simulink model "Assignment1"  (R2017a)
settings: Solver=FixedStepAuto  StartTime=0.0  StopTime=10.0  FixedStep=1E-3  RelTol=1e-3  EnableMultiTasking=on
undefined symbols (not defined in the file): D0, D1, D10, D11, D12, D13, D2, D3, D4, D5, D6, D7, D8, D9, PTA0, PTA1, PTA2, PTB23, PTB9, PTC16, PTC17, PTC2, PTC3, PTC4, PTD0, PTD1, PTD2, PTD3
libraries: frdmk64flib x18
settings Model: ExtModeTrigDuration=5  Creator=Nathe  LastModifiedBy=Nathe
settings DataIOCC: ReturnWorkspaceOutputs=on
settings OptimizationCC: EnhancedBackFolding=on  PassReuseOutputArgsAs=Individual arguments  ZeroExternalMemoryAtStartup=off  ZeroInternalMemoryAtStartup=off  MaxStackSize=64  OptimizeBlockOrder=speed
settings DebuggingCC: ParameterTunabilityLossMsg=error
settings HardwareCC: ProdBitPerPointer=32  ProdBitPerSizeT=32  ProdBitPerPtrDiffT=32  ProdLargestAtomicInteger=Long  ProdLargestAtomicFloat=Double  ProdWordSize=32  ProdHWDeviceType=ARM Compatible->ARM Cortex
settings SFSimCC: SimUseLocalCustomCode=on  MATLABDynamicMemAlloc=off
settings RTWCC: SystemTargetFile=ert.tlc  HardwareBoard=NXP FRDM-K64F  TLCOptions="-aInlineSetEventsForThisBaseRateFcn=TLC_FALSE -aSuppressMultiTaskScheduler=TLC_FALSE  -aRateBasedStepFcn=0"  TemplateMakefile=ert_default_tmf  Description=Embedded Coder  GenerateReport=on  RTWUseLocalCustomCode=on  Toolchain=GNU Tools for ARM Embedded Processors  IncludeHyperlinkInReport=on  LaunchReport=on  GenerateTraceInfo=on  GenerateTraceReport=on  GenerateTraceReportSl=on  GenerateTraceReportSf=on  GenerateTraceReportEml=on
settings CodeAppCC: ForceParamTrailComments=on  IgnoreCustomStorageClasses=off  OperatorAnnotations=on  SimulinkDataObjDesc=on  SFDataObjDesc=on  InsertBlockDesc=on
settings ERTTargetCC: SupportContinuousTime=on
settings SimscapeCC: SelectedTab=General

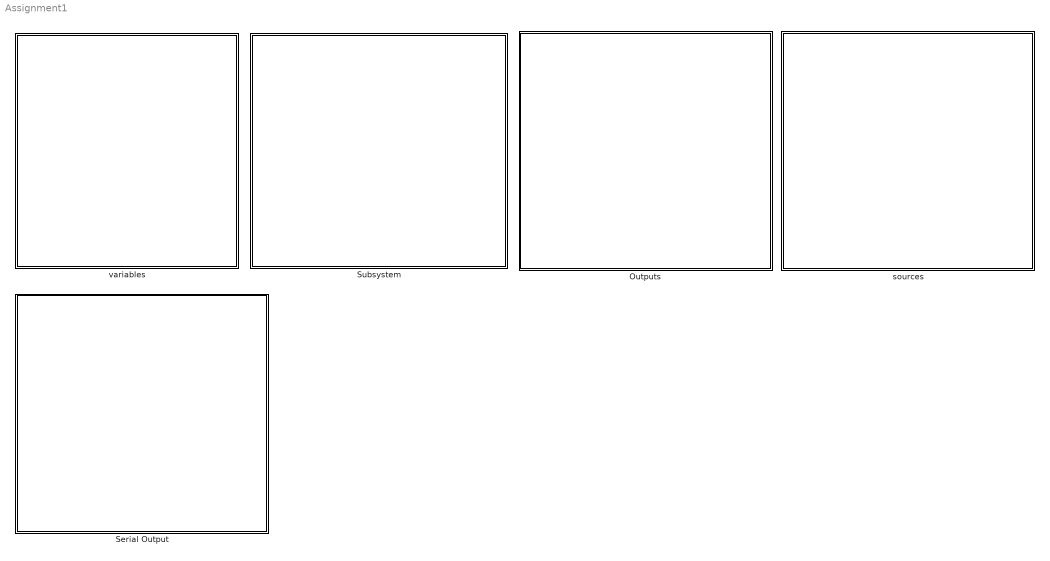
== system Assignment1 ==
  "Outputs " : Subsystem
  Serial Output : Subsystem
  Subsystem : Subsystem
  "sources " : Subsystem
  "variables " : Subsystem

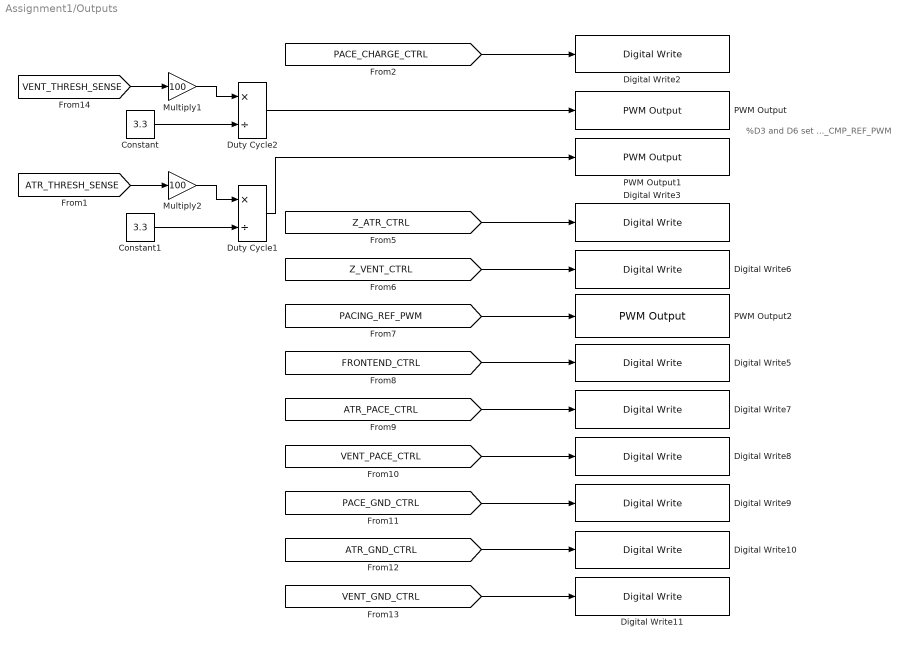
== system Assignment1/Outputs  ==
  note: %D3 and D6 set ..._CMP_REF_PWM
  Constant : Constant  Value=3.3
  Constant1 : Constant  Value=3.3
  Digital Write10 : frdmk64flib/Digital Write  Whichpin=PTD2 (D11)
      settings: SourceProductName=Simulink Coder Support Package for NXP FRDM-K64F Board
  Digital Write11 : frdmk64flib/Digital Write  Whichpin=PTD3 (D12)
      settings: SourceProductName=Simulink Coder Support Package for NXP FRDM-K64F Board
  Digital Write2 : frdmk64flib/Digital Write  Whichpin=PTB9 (D2)
      settings: SourceProductName=Simulink Coder Support Package for NXP FRDM-K64F Board
  Digital Write3 : frdmk64flib/Digital Write  Whichpin=PTB23 (D4)
      settings: SourceProductName=Simulink Coder Support Package for NXP FRDM-K64F Board
  Digital Write5 : frdmk64flib/Digital Write  Whichpin=PTD1 (D13)
      settings: SourceProductName=Simulink Coder Support Package for NXP FRDM-K64F Board
  Digital Write6 : frdmk64flib/Digital Write  Whichpin=PTC3 (D7)
      settings: SourceProductName=Simulink Coder Support Package for NXP FRDM-K64F Board
  Digital Write7 : frdmk64flib/Digital Write  Whichpin=PTA0 (D8)
      settings: SourceProductName=Simulink Coder Support Package for NXP FRDM-K64F Board
  Digital Write8 : frdmk64flib/Digital Write  Whichpin=PTC4 (D9)
      settings: SourceProductName=Simulink Coder Support Package for NXP FRDM-K64F Board
  Digital Write9 : frdmk64flib/Digital Write  Whichpin=PTD0 (D10)
      settings: SourceProductName=Simulink Coder Support Package for NXP FRDM-K64F Board
  Duty Cycle1 : Product  Inputs=*/  SaturateOnIntegerOverflow=off  RndMeth=Floor  InputSameDT=off  OutDataTypeStr=Inherit: Inherit via internal rule
  Duty Cycle2 : Product  Inputs=*/  SaturateOnIntegerOverflow=off  RndMeth=Floor  InputSameDT=off  OutDataTypeStr=Inherit: Inherit via internal rule
  Multiply1 : Gain  Gain=100
  Multiply2 : Gain  Gain=100
  PWM Output : frdmk64flib/PWM Output  Whichpin=PTA1 (D3)  InitialFrequency=2000  InitialDutyCycle=0
      settings: SourceProductName=Simulink Coder Support Package for NXP FRDM-K64F Board
  PWM Output1 : frdmk64flib/PWM Output  Whichpin=PTC2 (D6)  InitialFrequency=2000  InitialDutyCycle=0
      settings: SourceProductName=Simulink Coder Support Package for NXP FRDM-K64F Board
  PWM Output2 : frdmk64flib/PWM Output  Whichpin=PTA2 (D5)  InitialFrequency=2000  InitialDutyCycle=0
      settings: SourceProductName=Simulink Coder Support Package for NXP FRDM-K64F Board
  wires:
  [PACING_REF_PWM] -> PWM Output2/1
  [VENT_GND_CTRL] -> Digital Write11/1
  [PACE_GND_CTRL] -> Digital Write9/1
  [FRONTEND_CTRL] -> Digital Write5/1
  [VENT_PACE_CTRL] -> Digital Write8/1
  [ATR_PACE_CTRL] -> Digital Write7/1
  [Z_VENT_CTRL] -> Digital Write6/1
  [ATR_GND_CTRL] -> Digital Write10/1
  [PACE_CHARGE_CTRL] -> Digital Write2/1
  Duty Cycle2/1 -> PWM Output/1
  [Z_ATR_CTRL] -> Digital Write3/1
  [VENT_THRESH_SENSE] -> Multiply1/1
  Duty Cycle1/1 -> PWM Output1/1
  Constant1/1 -> Duty Cycle1/2
  Constant/1 -> Duty Cycle2/2
  [ATR_THRESH_SENSE] -> Multiply2/1
  Multiply1/1 -> Duty Cycle2/1
  Multiply2/1 -> Duty Cycle1/1

== system Assignment1/Serial Output ==

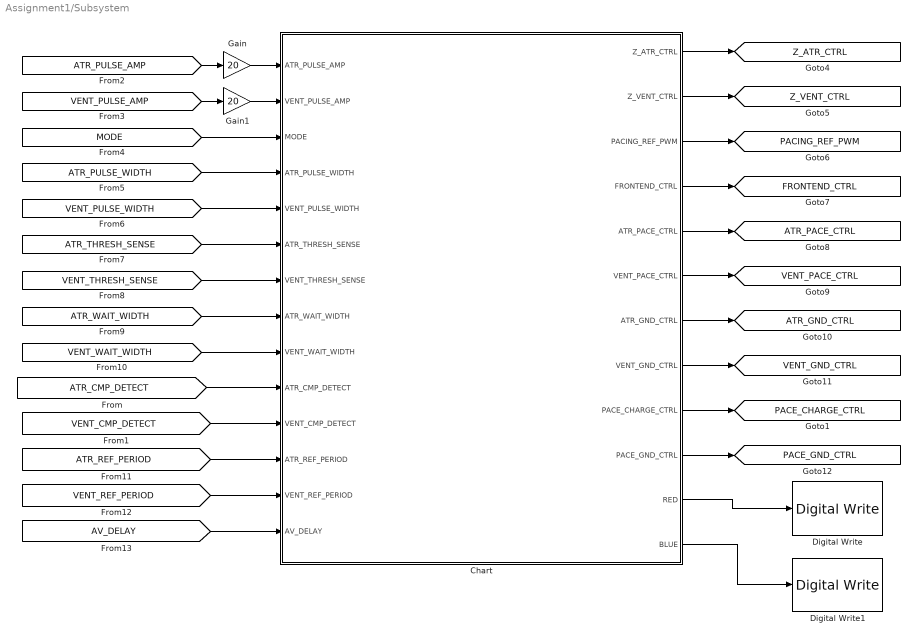
== system Assignment1/Subsystem ==
  Chart : Stateflow chart  TreatAsAtomicUnit=on
  Digital Write : frdmk64flib/Digital Write  Whichpin=RED_LED
      settings: SourceProductName=Simulink Coder Support Package for NXP FRDM-K64F Board
  Digital Write1 : frdmk64flib/Digital Write  Whichpin=BLUE_LED
      settings: SourceProductName=Simulink Coder Support Package for NXP FRDM-K64F Board
  Gain : Gain  Gain=20
  Gain1 : Gain  Gain=20
  tag scope: ATR_GND_CTRL=global, ATR_PACE_CTRL=global, FRONTEND_CTRL=global, PACE_CHARGE_CTRL=global, PACE_GND_CTRL=global, PACING_REF_PWM=global, VENT_GND_CTRL=global, VENT_PACE_CTRL=global, Z_ATR_CTRL=global, Z_VENT_CTRL=global
  wires:
  [ATR_CMP_DETECT] -> Chart/10(ATR_CMP_DETECT)
  Gain/1 -> Chart/1(ATR_PULSE_AMP)
  Chart/3(PACING_REF_PWM) -> [PACING_REF_PWM]
  Chart/7(ATR_GND_CTRL) -> [ATR_GND_CTRL]
  [VENT_WAIT_WIDTH] -> Chart/9(VENT_WAIT_WIDTH)
  Chart/2(Z_VENT_CTRL) -> [Z_VENT_CTRL]
  Chart/5(ATR_PACE_CTRL) -> [ATR_PACE_CTRL]
  [VENT_PULSE_WIDTH] -> Chart/5(VENT_PULSE_WIDTH)
  [ATR_PULSE_AMP] -> Gain/1
  Chart/9(PACE_CHARGE_CTRL) -> [PACE_CHARGE_CTRL]
  [ATR_PULSE_WIDTH] -> Chart/4(ATR_PULSE_WIDTH)
  Chart/8(VENT_GND_CTRL) -> [VENT_GND_CTRL]
  Chart/1(Z_ATR_CTRL) -> [Z_ATR_CTRL]
  [VENT_PULSE_AMP] -> Gain1/1
  [VENT_THRESH_SENSE] -> Chart/7(VENT_THRESH_SENSE)
  [VENT_CMP_DETECT] -> Chart/11(VENT_CMP_DETECT)
  Chart/4(FRONTEND_CTRL) -> [FRONTEND_CTRL]
  Chart/6(VENT_PACE_CTRL) -> [VENT_PACE_CTRL]
  [MODE] -> Chart/3(MODE)
  [ATR_THRESH_SENSE] -> Chart/6(ATR_THRESH_SENSE)
  [ATR_WAIT_WIDTH] -> Chart/8(ATR_WAIT_WIDTH)
  Gain1/1 -> Chart/2(VENT_PULSE_AMP)
  Chart/10(PACE_GND_CTRL) -> [PACE_GND_CTRL]
  Chart/11(RED) -> Digital Write/1
  Chart/12(BLUE) -> Digital Write1/1
  [ATR_REF_PERIOD] -> Chart/12(ATR_REF_PERIOD)
  [VENT_REF_PERIOD] -> Chart/13(VENT_REF_PERIOD)
  [AV_DELAY] -> Chart/14(AV_DELAY)

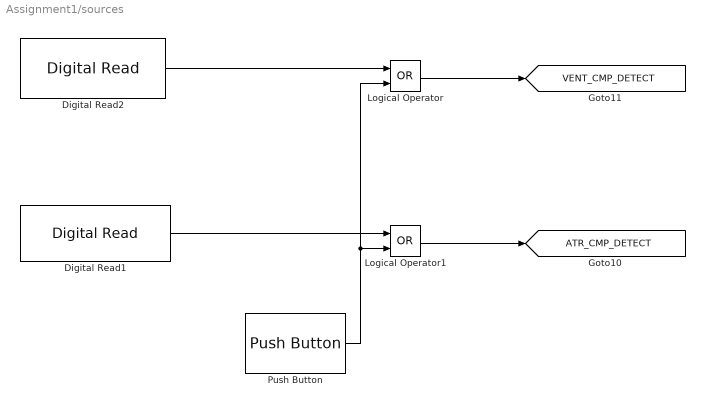
== system Assignment1/sources  ==
  Digital Read1 : frdmk64flib/Digital Read  Whichpin=PTC16 (D0)  SampleTime=-1
      settings: SourceProductName=Simulink Coder Support Package for NXP FRDM-K64F Board
  Digital Read2 : frdmk64flib/Digital Read  Whichpin=PTC17 (D1)  SampleTime=-1
      settings: SourceProductName=Simulink Coder Support Package for NXP FRDM-K64F Board
  Logical Operator : Logic  Operator=OR  AllPortsSameDT=off  OutDataTypeStr=boolean
  Logical Operator1 : Logic  Operator=OR  AllPortsSameDT=off  OutDataTypeStr=boolean
  Push Button : frdmk64flib/Push Button  Whichswitch=SW2  SampleTime1=-1
      settings: SourceProductName=Simulink Coder Support Package for NXP FRDM-K64F Board
  tag scope: ATR_CMP_DETECT=global, VENT_CMP_DETECT=global
  wires:
  Digital Read2/1 -> Logical Operator/1
  Logical Operator/1 -> [VENT_CMP_DETECT]
  Digital Read1/1 -> Logical Operator1/1
  Logical Operator1/1 -> [ATR_CMP_DETECT]
  Push Button/1 -> Logical Operator/2, Logical Operator1/2

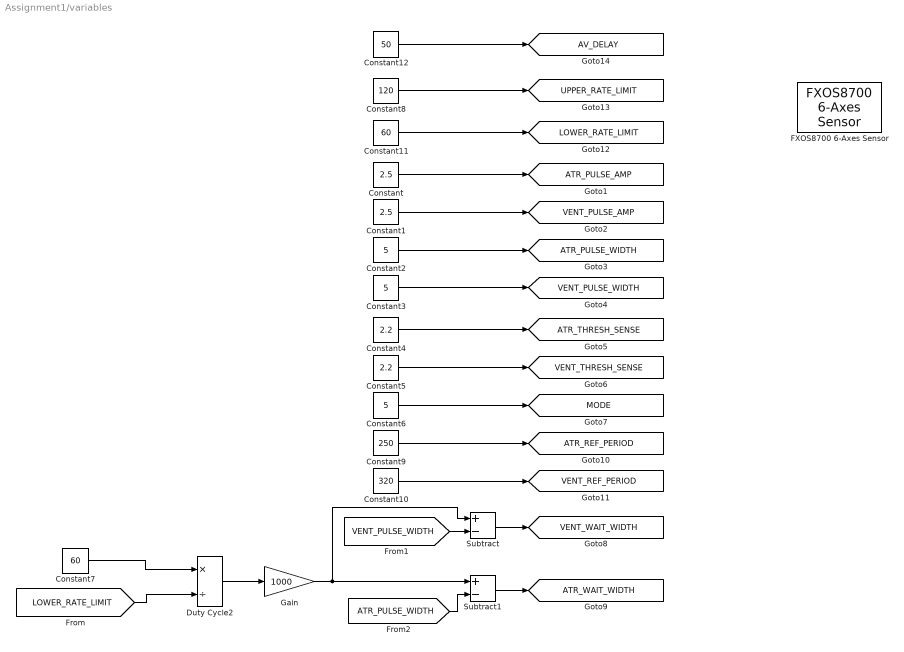
== system Assignment1/variables  ==
  Constant : Constant  Value=2.5
  Constant1 : Constant  Value=2.5
  Constant10 : Constant  Value=320
  Constant11 : Constant  Value=60
  Constant12 : Constant  Value=50
  Constant2 : Constant  Value=5
  Constant3 : Constant  Value=5
  Constant4 : Constant  Value=2.2
  Constant5 : Constant  Value=2.2
  Constant6 : Constant  Value=5  OutDataTypeStr=int8
  Constant7 : Constant  Value=60
  Constant8 : Constant  Value=120
  Constant9 : Constant  Value=250
  Duty Cycle2 : Product  Inputs=*/  SaturateOnIntegerOverflow=off  RndMeth=Floor  InputSameDT=off  OutDataTypeStr=Inherit: Inherit via internal rule
  FXOS8700 6-Axes Sensor : frdmk64flib/FXOS8700 6-Axes Sensor  Activesensor=Accelerometer only  ODR=800Hz  HybridODR=400Hz  Accelfullrange=-4g to +4g  SampleTime=-1
      settings: SourceProductName=Simulink Coder Support Package for NXP FRDM-K64F Board
  Gain : Gain  Gain=1000
  Subtract : Sum  Inputs=+-  SaturateOnIntegerOverflow=off  InputSameDT=off  OutDataTypeStr=Inherit: Inherit via internal rule
  Subtract1 : Sum  Inputs=+-  SaturateOnIntegerOverflow=off  InputSameDT=off  OutDataTypeStr=Inherit: Inherit via internal rule
  tag scope: ATR_PULSE_AMP=global, ATR_PULSE_WIDTH=global, ATR_REF_PERIOD=global, ATR_THRESH_SENSE=global, ATR_WAIT_WIDTH=global, AV_DELAY=global, LOWER_RATE_LIMIT=global, MODE=global, UPPER_RATE_LIMIT=global, VENT_PULSE_AMP=global, VENT_PULSE_WIDTH=global, VENT_REF_PERIOD=global, VENT_THRESH_SENSE=global, VENT_WAIT_WIDTH=global
  wires:
  Constant3/1 -> [VENT_PULSE_WIDTH]
  Constant2/1 -> [ATR_PULSE_WIDTH]
  Constant/1 -> [ATR_PULSE_AMP]
  Constant5/1 -> [VENT_THRESH_SENSE]
  Constant1/1 -> [VENT_PULSE_AMP]
  Constant4/1 -> [ATR_THRESH_SENSE]
  Constant6/1 -> [MODE]
  Subtract/1 -> [VENT_WAIT_WIDTH]
  Subtract1/1 -> [ATR_WAIT_WIDTH]
  Constant9/1 -> [ATR_REF_PERIOD]
  Constant10/1 -> [VENT_REF_PERIOD]
  Constant11/1 -> [LOWER_RATE_LIMIT]
  Constant7/1 -> Duty Cycle2/1
  [LOWER_RATE_LIMIT] -> Duty Cycle2/2
  Duty Cycle2/1 -> Gain/1
  Gain/1 -> Subtract1/1, Subtract/1
  [VENT_PULSE_WIDTH] -> Subtract/2
  [ATR_PULSE_WIDTH] -> Subtract1/2
  Constant8/1 -> [UPPER_RATE_LIMIT]
  Constant12/1 -> [AV_DELAY]

== stateflow chart Assignment1/Subsystem/Chart ==
  state AAIR [group]
    state CHARGEC22_DISCHARGEC21
      during:
      %CHARGE C22
      PACING_REF_PWM = ATR_PULSE_AMP
      PACE_CHARGE_CTRL = true
      ATR_PACE_CTRL = false
      VENT_PACE_CTRL = false
      %DISCHARGE C21
      PACE_GND_CTRL = true
      VENT_PACE_CTRL = false
      VENT_GND_CTRL = false
      ATR_GND_CTRL = true
      RED = false
      BLUE = false
      Z_ATR_CTRL=false
      Z_VENT_CTRL=false
      FRONTEND_CTRL=true
    state DISCHARGEC22
      %paces atrium
      during:
      %CHARGE C21
      ATR_PACE_CTRL = true
      PACE_CHARGE_CTRL = false
      ATR_GND_CTRL = false
      PACE_GND_CTRL = true
      VENT_PACE_CTRL = false
      VENT_GND_CTRL = false
      Z_ATR_CTRL=false
      Z_VENT_CTRL=false
      FRONTEND_CTRL=true
      RED = true
    state CHARGEC22_DISCHARGEC21_2
      during:
      %CHARGE C22
      PACING_REF_PWM = ATR_PULSE_AMP
      PACE_CHARGE_CTRL = true
      ATR_PACE_CTRL = false
      VENT_PACE_CTRL = false
      %DISCHARGE C21
      PACE_GND_CTRL = true
      VENT_PACE_CTRL = false
      VENT_GND_CTRL = false
      ATR_GND_CTRL = true
      RED = false
      BLUE = false
      Z_ATR_CTRL=false
      Z_VENT_CTRL=false
      FRONTEND_CTRL=true
    state DUMMY
      during:
      BLUE = true
      RED = false
    AAIR.CHARGEC22_DISCHARGEC21 -> AAIR.DISCHARGEC22 [order 1] : after(ATR_WAIT_WIDTH - ATR_REF_PERIOD, msec)
    AAIR.CHARGEC22_DISCHARGEC21_2 -> AAIR.CHARGEC22_DISCHARGEC21 [order 1] : after(ATR_REF_PERIOD, msec)
    AAIR.DISCHARGEC22 -> AAIR.CHARGEC22_DISCHARGEC21_2 : after(ATR_PULSE_WIDTH, msec)
    AAIR.DUMMY -> AAIR.CHARGEC22_DISCHARGEC21 : after(ATR_REF_PERIOD, msec)
    AAIR.CHARGEC22_DISCHARGEC21 -> AAIR.DUMMY [order 2] : [ATR_CMP_DETECT == true]
    AAIR.CHARGEC22_DISCHARGEC21_2 -> AAIR.DUMMY [order 2] : [ATR_CMP_DETECT == true]
  state AOOR [group]
    state CHARGEC22_DISCHARGEC21
      during:
      %CHARGE C22
      PACING_REF_PWM = ATR_PULSE_AMP
      PACE_CHARGE_CTRL = true
      ATR_PACE_CTRL = false
      VENT_PACE_CTRL = false
      %DISCHARGE C21
      PACE_GND_CTRL = true
      VENT_PACE_CTRL = false
      VENT_GND_CTRL = false
      ATR_GND_CTRL = true
      Z_ATR_CTRL=false
      Z_VENT_CTRL=false
      FRONTEND_CTRL=true
      RED = false
    state DISCHARGEC22
      %paces atrium
      during:
      %CHARGE C21
      ATR_PACE_CTRL = true
      PACE_CHARGE_CTRL = false
      ATR_GND_CTRL = false
      PACE_GND_CTRL = true
      VENT_PACE_CTRL = false
      VENT_GND_CTRL = false
      Z_ATR_CTRL=false
      Z_VENT_CTRL=false
      FRONTEND_CTRL=true
      RED = true
    AOOR.CHARGEC22_DISCHARGEC21 -> AOOR.DISCHARGEC22 : after(ATR_WAIT_WIDTH, msec)
    AOOR.DISCHARGEC22 -> AOOR.CHARGEC22_DISCHARGEC21 : after(ATR_PULSE_WIDTH, msec)
  state DOOR [group]
    state DISCHARGEC22
      %paces atrium
      during:
      %CHARGE C21
      ATR_PACE_CTRL = true
      PACE_CHARGE_CTRL = false
      ATR_GND_CTRL = false
      PACE_GND_CTRL = true
      VENT_PACE_CTRL = false
      VENT_GND_CTRL = false
      Z_ATR_CTRL=false
      Z_VENT_CTRL=false
      FRONTEND_CTRL=true
      RED = true
    state CHARGEC22_DISCHARGEC21
      during:
      %CHARGE C22
      PACING_REF_PWM = ATR_PULSE_AMP
      PACE_CHARGE_CTRL = true
      ATR_PACE_CTRL = false
      VENT_PACE_CTRL = false
      %DISCHARGE C21
      PACE_GND_CTRL = true
      VENT_GND_CTRL = true
      ATR_GND_CTRL = false
      Z_ATR_CTRL=false
      Z_VENT_CTRL=false
      FRONTEND_CTRL=true
      BLUE = false
    state CHARGEC22_DISCHARGEC22
      during:
      %CHARGE C22
      PACING_REF_PWM = VENT_PULSE_AMP
      PACE_CHARGE_CTRL= true
      ATR_PACE_CTRL = false
      VENT_PACE_CTRL = false
      %DISCHARGE C21
      PACE_GND_CTRL = true
      VENT_GND_CTRL = false
      ATR_GND_CTRL = true
      Z_ATR_CTRL=false
      Z_VENT_CTRL=false
      FRONTEND_CTRL=true
      RED = false
    state DISCHARGEC21
      %pacing through ventricle
      during:
      %CHARGING C21 & DISCHARGING C22
      VENT_PACE_CTRL = true
      PACE_CHARGE_CTRL = false
      VENT_GND_CTRL = false
      PACE_GND_CTRL = true
      ATR_PACE_CTRL = false
      ATR_GND_CTRL = false
      Z_ATR_CTRL=false
      Z_VENT_CTRL=false
      FRONTEND_CTRL=true
      BLUE = true
    DOOR.CHARGEC22_DISCHARGEC21 -> DOOR.DISCHARGEC22 : after(VENT_WAIT_WIDTH - AV_DELAY, msec)
    DOOR.DISCHARGEC22 -> DOOR.CHARGEC22_DISCHARGEC22 : after(ATR_PULSE_WIDTH, msec)
    DOOR.DISCHARGEC21 -> DOOR.CHARGEC22_DISCHARGEC21 : after(VENT_PULSE_WIDTH, msec)
    DOOR.CHARGEC22_DISCHARGEC22 -> DOOR.DISCHARGEC21 : after(AV_DELAY - ATR_PULSE_WIDTH, msec)
  state VVIR [group]
    state CHARGEC22_DISCHARGEC21
      during:
      %CHARGE C22
      PACING_REF_PWM = VENT_PULSE_AMP
      PACE_CHARGE_CTRL = true
      VENT_PACE_CTRL = false
      ATR_PACE_CTRL = false
      %DISCHARGE C21
      PACE_GND_CTRL = true
      ATR_PACE_CTRL = false
      ATR_GND_CTRL = false
      VENT_GND_CTRL = true
      RED = false
      BLUE = false
      Z_ATR_CTRL=false
      Z_VENT_CTRL=false
      FRONTEND_CTRL=true
    state DISCHARGEC22
      %paces vent
      during:
      %CHARGE C21
      VENT_PACE_CTRL = true
      PACE_CHARGE_CTRL = false
      VENT_GND_CTRL = false
      PACE_GND_CTRL = true
      ATR_PACE_CTRL = false
      ATR_GND_CTRL = false
      Z_ATR_CTRL=false
      Z_VENT_CTRL=false
      FRONTEND_CTRL=true
      RED = true
      BLUE = false
    state CHARGEC22_DISCHARGEC21_2
      during:
      %CHARGE C22
      PACING_REF_PWM = VENT_PULSE_AMP
      PACE_CHARGE_CTRL = true
      VENT_PACE_CTRL = false
      ATR_PACE_CTRL = false
      %DISCHARGE C21
      PACE_GND_CTRL = true
      ATR_PACE_CTRL = false
      ATR_GND_CTRL = false
      VENT_GND_CTRL = true
      RED = false
      BLUE = false
      Z_ATR_CTRL=false
      Z_VENT_CTRL=false
      FRONTEND_CTRL=true
    state DUMMY
      during:
      BLUE = true
      RED = false
    VVIR.CHARGEC22_DISCHARGEC21 -> VVIR.DISCHARGEC22 [order 1] : after(VENT_WAIT_WIDTH - VENT_REF_PERIOD, msec)
    VVIR.CHARGEC22_DISCHARGEC21_2 -> VVIR.CHARGEC22_DISCHARGEC21 [order 1] : after(VENT_REF_PERIOD, msec)
    VVIR.DISCHARGEC22 -> VVIR.CHARGEC22_DISCHARGEC21_2 : after(VENT_PULSE_WIDTH, msec)
    VVIR.DUMMY -> VVIR.CHARGEC22_DISCHARGEC21 : after(VENT_REF_PERIOD, msec)
    VVIR.CHARGEC22_DISCHARGEC21 -> VVIR.DUMMY [order 2] : [VENT_CMP_DETECT == true]
    VVIR.CHARGEC22_DISCHARGEC21_2 -> VVIR.DUMMY [order 2] : [VENT_CMP_DETECT == true]
  state VOOR [group]
    state CHARGEC22_DISCHARGEC21
      during:
      %CHARGE C22
      PACING_REF_PWM = VENT_PULSE_AMP
      PACE_CHARGE_CTRL= true
      ATR_PACE_CTRL = false
      VENT_PACE_CTRL = false
      %DISCHARGING C21
      PACE_GND_CTRL = true
      VENT_PACE_CTRL = false
      ATR_GND_CTRL = false
      VENT_GND_CTRL = true
      Z_ATR_CTRL=false
      Z_VENT_CTRL=false
      FRONTEND_CTRL=true
      RED = false
    state DISCHARGEC22
      %pacing through ventricle
      during:
      %CHARGING C21 & DISCHARGING C22
      VENT_PACE_CTRL = true
      PACE_CHARGE_CTRL = false
      VENT_GND_CTRL = false
      PACE_GND_CTRL = true
      ATR_PACE_CTRL = false
      ATR_GND_CTRL = false
      Z_ATR_CTRL=false
      Z_VENT_CTRL=false
      FRONTEND_CTRL=true
      RED = true
    VOOR.CHARGEC22_DISCHARGEC21 -> VOOR.DISCHARGEC22 : after(VENT_WAIT_WIDTH, msec)
    VOOR.DISCHARGEC22 -> VOOR.CHARGEC22_DISCHARGEC21 : after(VENT_PULSE_WIDTH, msec)
  state START_HERE
  state AAI [group]
    state CHARGEC22_DISCHARGEC21
      during:
      %CHARGE C22
      PACING_REF_PWM = ATR_PULSE_AMP
      PACE_CHARGE_CTRL = true
      ATR_PACE_CTRL = false
      VENT_PACE_CTRL = false
      %DISCHARGE C21
      PACE_GND_CTRL = true
      VENT_PACE_CTRL = false
      VENT_GND_CTRL = false
      ATR_GND_CTRL = true
      RED = false
      BLUE = false
      Z_ATR_CTRL=false
      Z_VENT_CTRL=false
      FRONTEND_CTRL=true
    state DISCHARGEC22
      %paces atrium
      during:
      %CHARGE C21
      ATR_PACE_CTRL = true
      PACE_CHARGE_CTRL = false
      ATR_GND_CTRL = false
      PACE_GND_CTRL = true
      VENT_PACE_CTRL = false
      VENT_GND_CTRL = false
      Z_ATR_CTRL=false
      Z_VENT_CTRL=false
      FRONTEND_CTRL=true
      RED = true
    state CHARGEC22_DISCHARGEC21_2
      during:
      %CHARGE C22
      PACING_REF_PWM = ATR_PULSE_AMP
      PACE_CHARGE_CTRL = true
      ATR_PACE_CTRL = false
      VENT_PACE_CTRL = false
      %DISCHARGE C21
      PACE_GND_CTRL = true
      VENT_PACE_CTRL = false
      VENT_GND_CTRL = false
      ATR_GND_CTRL = true
      RED = false
      BLUE = false
      Z_ATR_CTRL=false
      Z_VENT_CTRL=false
      FRONTEND_CTRL=true
    state DUMMY
      during:
      BLUE = true
      RED = false
    AAI.CHARGEC22_DISCHARGEC21 -> AAI.DISCHARGEC22 [order 1] : after(ATR_WAIT_WIDTH - ATR_REF_PERIOD, msec)
    AAI.CHARGEC22_DISCHARGEC21_2 -> AAI.CHARGEC22_DISCHARGEC21 [order 1] : after(ATR_REF_PERIOD, msec)
    AAI.DISCHARGEC22 -> AAI.CHARGEC22_DISCHARGEC21_2 : after(ATR_PULSE_WIDTH, msec)
    AAI.DUMMY -> AAI.CHARGEC22_DISCHARGEC21 : after(ATR_REF_PERIOD, msec)
    AAI.CHARGEC22_DISCHARGEC21 -> AAI.DUMMY [order 2] : [ATR_CMP_DETECT == true]
    AAI.CHARGEC22_DISCHARGEC21_2 -> AAI.DUMMY [order 2] : [ATR_CMP_DETECT == true]
  state AOO [group]
    state CHARGEC22_DISCHARGEC21
      during:
      %CHARGE C22
      PACING_REF_PWM = ATR_PULSE_AMP
      PACE_CHARGE_CTRL = true
      ATR_PACE_CTRL = false
      VENT_PACE_CTRL = false
      %DISCHARGE C21
      PACE_GND_CTRL = true
      VENT_PACE_CTRL = false
      VENT_GND_CTRL = false
      ATR_GND_CTRL = true
      Z_ATR_CTRL=false
      Z_VENT_CTRL=false
      FRONTEND_CTRL=true
      RED = false
    state DISCHARGEC22
      %paces atrium
      during:
      %CHARGE C21
      ATR_PACE_CTRL = true
      PACE_CHARGE_CTRL = false
      ATR_GND_CTRL = false
      PACE_GND_CTRL = true
      VENT_PACE_CTRL = false
      VENT_GND_CTRL = false
      Z_ATR_CTRL=false
      Z_VENT_CTRL=false
      FRONTEND_CTRL=true
      RED = true
    AOO.CHARGEC22_DISCHARGEC21 -> AOO.DISCHARGEC22 : after(ATR_WAIT_WIDTH, msec)
    AOO.DISCHARGEC22 -> AOO.CHARGEC22_DISCHARGEC21 : after(ATR_PULSE_WIDTH, msec)
  state DOO [group]
    state DISCHARGEC22
      %paces atrium
      during:
      %CHARGE C21
      ATR_PACE_CTRL = true
      PACE_CHARGE_CTRL = false
      ATR_GND_CTRL = false
      PACE_GND_CTRL = true
      VENT_PACE_CTRL = false
      VENT_GND_CTRL = false
      Z_ATR_CTRL=false
      Z_VENT_CTRL=false
      FRONTEND_CTRL=true
      RED = true
    state CHARGEC22_DISCHARGEC21
      during:
      %CHARGE C22
      PACING_REF_PWM = ATR_PULSE_AMP
      PACE_CHARGE_CTRL = true
      ATR_PACE_CTRL = false
      VENT_PACE_CTRL = false
      %DISCHARGE C21
      PACE_GND_CTRL = true
      VENT_GND_CTRL = true
      ATR_GND_CTRL = false
      Z_ATR_CTRL=false
      Z_VENT_CTRL=false
      FRONTEND_CTRL=true
      BLUE = false
    state CHARGEC22_DISCHARGEC22
      during:
      %CHARGE C22
      PACING_REF_PWM = VENT_PULSE_AMP
      PACE_CHARGE_CTRL= true
      ATR_PACE_CTRL = false
      VENT_PACE_CTRL = false
      %DISCHARGE C21
      PACE_GND_CTRL = true
      VENT_GND_CTRL = false
      ATR_GND_CTRL = true
      Z_ATR_CTRL=false
      Z_VENT_CTRL=false
      FRONTEND_CTRL=true
      RED = false
    state DISCHARGEC21
      %pacing through ventricle
      during:
      %CHARGING C21 & DISCHARGING C22
      VENT_PACE_CTRL = true
      PACE_CHARGE_CTRL = false
      VENT_GND_CTRL = false
      PACE_GND_CTRL = true
      ATR_PACE_CTRL = false
      ATR_GND_CTRL = false
      Z_ATR_CTRL=false
      Z_VENT_CTRL=false
      FRONTEND_CTRL=true
      BLUE = true
    DOO.CHARGEC22_DISCHARGEC21 -> DOO.DISCHARGEC22 : after(VENT_WAIT_WIDTH - AV_DELAY, msec)
    DOO.DISCHARGEC22 -> DOO.CHARGEC22_DISCHARGEC22 : after(ATR_PULSE_WIDTH, msec)
    DOO.DISCHARGEC21 -> DOO.CHARGEC22_DISCHARGEC21 : after(VENT_PULSE_WIDTH, msec)
    DOO.CHARGEC22_DISCHARGEC22 -> DOO.DISCHARGEC21 : after(AV_DELAY - ATR_PULSE_WIDTH, msec)
  state VVI [group]
    state CHARGEC22_DISCHARGEC21
      during:
      %CHARGE C22
      PACING_REF_PWM = VENT_PULSE_AMP
      PACE_CHARGE_CTRL = true
      VENT_PACE_CTRL = false
      ATR_PACE_CTRL = false
      %DISCHARGE C21
      PACE_GND_CTRL = true
      ATR_PACE_CTRL = false
      ATR_GND_CTRL = false
      VENT_GND_CTRL = true
      RED = false
      BLUE = false
      Z_ATR_CTRL=false
      Z_VENT_CTRL=false
      FRONTEND_CTRL=true
    state DISCHARGEC22
      %paces vent
      during:
      %CHARGE C21
      VENT_PACE_CTRL = true
      PACE_CHARGE_CTRL = false
      VENT_GND_CTRL = false
      PACE_GND_CTRL = true
      ATR_PACE_CTRL = false
      ATR_GND_CTRL = false
      Z_ATR_CTRL=false
      Z_VENT_CTRL=false
      FRONTEND_CTRL=true
      RED = true
      BLUE = false
    state CHARGEC22_DISCHARGEC21_2
      during:
      %CHARGE C22
      PACING_REF_PWM = VENT_PULSE_AMP
      PACE_CHARGE_CTRL = true
      VENT_PACE_CTRL = false
      ATR_PACE_CTRL = false
      %DISCHARGE C21
      PACE_GND_CTRL = true
      ATR_PACE_CTRL = false
      ATR_GND_CTRL = false
      VENT_GND_CTRL = true
      RED = false
      BLUE = false
      Z_ATR_CTRL=false
      Z_VENT_CTRL=false
      FRONTEND_CTRL=true
    state DUMMY
      during:
      BLUE = true
      RED = false
    VVI.CHARGEC22_DISCHARGEC21 -> VVI.DISCHARGEC22 [order 1] : after(VENT_WAIT_WIDTH - VENT_REF_PERIOD, msec)
    VVI.CHARGEC22_DISCHARGEC21_2 -> VVI.CHARGEC22_DISCHARGEC21 [order 1] : after(VENT_REF_PERIOD, msec)
    VVI.DISCHARGEC22 -> VVI.CHARGEC22_DISCHARGEC21_2 : after(VENT_PULSE_WIDTH, msec)
    VVI.DUMMY -> VVI.CHARGEC22_DISCHARGEC21 : after(VENT_REF_PERIOD, msec)
    VVI.CHARGEC22_DISCHARGEC21 -> VVI.DUMMY [order 2] : [VENT_CMP_DETECT == true]
    VVI.CHARGEC22_DISCHARGEC21_2 -> VVI.DUMMY [order 2] : [VENT_CMP_DETECT == true]
  state VOO [group]
    state CHARGEC22_DISCHARGEC21
      during:
      %CHARGE C22
      PACING_REF_PWM = VENT_PULSE_AMP
      PACE_CHARGE_CTRL= true
      ATR_PACE_CTRL = false
      VENT_PACE_CTRL = false
      %DISCHARGING C21
      PACE_GND_CTRL = true
      VENT_PACE_CTRL = false
      ATR_GND_CTRL = false
      VENT_GND_CTRL = true
      Z_ATR_CTRL=false
      Z_VENT_CTRL=false
      FRONTEND_CTRL=true
      RED = false
    state DISCHARGEC22
      %pacing through ventricle
      during:
      %CHARGING C21 & DISCHARGING C22
      VENT_PACE_CTRL = true
      PACE_CHARGE_CTRL = false
      VENT_GND_CTRL = false
      PACE_GND_CTRL = true
      ATR_PACE_CTRL = false
      ATR_GND_CTRL = false
      Z_ATR_CTRL=false
      Z_VENT_CTRL=false
      FRONTEND_CTRL=true
      RED = true
    VOO.CHARGEC22_DISCHARGEC21 -> VOO.DISCHARGEC22 : after(VENT_WAIT_WIDTH, msec)
    VOO.DISCHARGEC22 -> VOO.CHARGEC22_DISCHARGEC21 : after(VENT_PULSE_WIDTH, msec)
  START_HERE -> AAIR.CHARGEC22_DISCHARGEC21 [order 7] : [MODE == 8]
  START_HERE -> DOOR.CHARGEC22_DISCHARGEC21 [order 8] : [MODE == 10]
  START_HERE -> VVIR.CHARGEC22_DISCHARGEC21 [order 9] : [MODE == 9]
  START_HERE -> AOOR.CHARGEC22_DISCHARGEC21 [order 6] : [MODE == 6]
  START_HERE -> VOOR.CHARGEC22_DISCHARGEC21 [order 10] : [MODE == 7]
  (default) -> START_HERE
  START_HERE -> DOO.CHARGEC22_DISCHARGEC21 [order 2] : [MODE == 5]
  START_HERE -> AAI.CHARGEC22_DISCHARGEC21 [order 5] : [MODE == 3]
  START_HERE -> VVI.CHARGEC22_DISCHARGEC21 [order 4] : [MODE == 4]
  START_HERE -> VOO.CHARGEC22_DISCHARGEC21 [order 3] : [MODE == 2]
  START_HERE -> AOO.CHARGEC22_DISCHARGEC21 [order 1] : [MODE == 1]
  data: ATR_PULSE_AMP input; VENT_PULSE_AMP input; MODE input int8; ATR_PULSE_WIDTH input; VENT_PULSE_WIDTH input; ATR_THRESH_SENSE input; VENT_THRESH_SENSE input; ATR_WAIT_WIDTH input; VENT_WAIT_WIDTH input; ATR_CMP_DETECT input boolean; VENT_CMP_DETECT input boolean; Z_ATR_CTRL output; Z_VENT_CTRL output; PACING_REF_PWM output; FRONTEND_CTRL output; ATR_PACE_CTRL output; VENT_PACE_CTRL output; ATR_GND_CTRL output; VENT_GND_CTRL output; PACE_CHARGE_CTRL output; PACE_GND_CTRL output; RED output; BLUE output; ATR_REF_PERIOD input; VENT_REF_PERIOD input; PB3 local; AV_DELAY input
